simulink model "FAM_simple_lab_scale_ref"  (R2023b)
settings: Solver=VariableStepAuto  StartTime=0.0  StopTime=10.0  MaxStep=0.01  RelTol=1e-3
libraries: FAM_simple_lab_scale x1
settings Model: Creator=Carson  LastModifiedBy=Carson

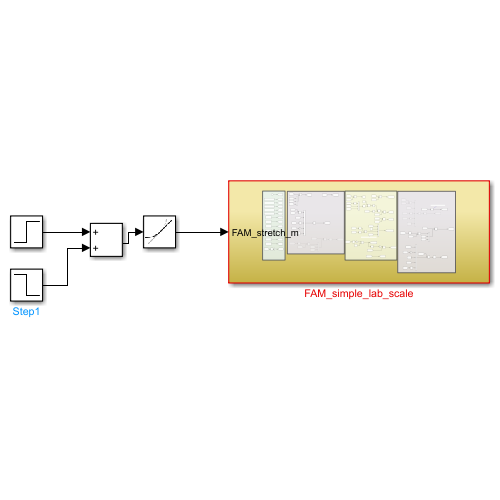
[thumbnail: Simulink's stored preview of the top-level diagram]
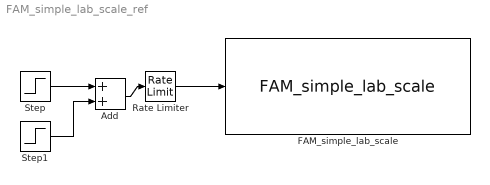
== system FAM_simple_lab_scale_ref ==
  Add : Sum
  FAM_simple_lab_scale : FAM_simple_lab_scale/FAM_simple_lab_scale  SystemSampleTime=-1  VariantActivationTime=update diagram  AllowFlexibleInterface=on  Latency=0  AutoFrameSizeCalculation=off
  Rate Limiter : RateLimiter  RisingSlewLimit=0.01  FallingSlewLimit=-0.01  SampleTimeMode=inherited
  Step : Step  After=0.025  SampleTime=0  ZeroCross=off
  Step1 : Step  Time=5  After=-0.025  SampleTime=0  ZeroCross=off
  wires:
  Rate Limiter/1 -> FAM_simple_lab_scale/1
  Step/1 -> Add/1
  Add/1 -> Rate Limiter/1
  Step1/1 -> Add/2
